simulink model "business"  (R2012b)
settings: Solver=ode3  StartTime=0.0  StopTime=10.0  FixedStep=1  RelTol=1e-3
settings Model: Creator=ägarenn  LastModifiedBy=ägarenn
settings OptimizationCC: InlineParams=on
settings DebuggingCC: SolverPrmCheckMsg=none

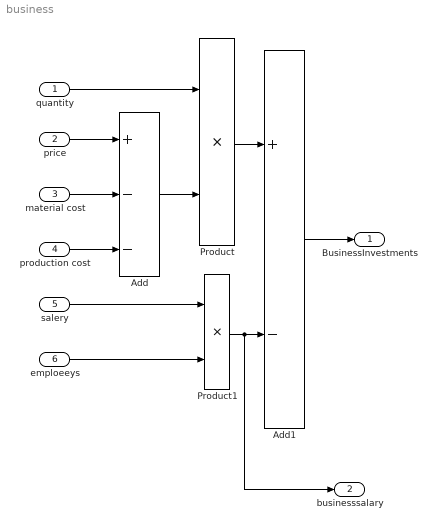
== system business ==
  quantity : Inport
  price : Inport  Port=2
  material cost : Inport  Port=3
  production cost : Inport  Port=4
  salery : Inport  Port=5
  emploeeys : Inport  Port=6
  Add : Sum  Inputs=+--
  Add1 : Sum  Inputs=+-
  Product : Product  RndMeth=Zero
  Product1 : Product  RndMeth=Zero
  BusinessInvestments : Outport
  businesssalary : Outport  Port=2
  wires:
  quantity/1 -> Product/1
  emploeeys/1 -> Product1/2
  salery/1 -> Product1/1
  production cost/1 -> Add/3
  price/1 -> Add/1
  material cost/1 -> Add/2
  Add/1 -> Product/2
  Product/1 -> Add1/1
  Product1/1 -> businesssalary/1, Add1/2
  Add1/1 -> BusinessInvestments/1
